simulink model "ariClinderSys"  (R2018a)
settings: Solver=VariableStepAuto  StartTime=0.0  StopTime=10.0  RelTol=1e-3
settings Model: Creator=wangmt  LastModifiedBy=wangmt

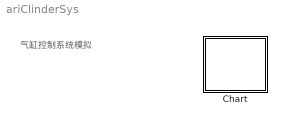
== system ariClinderSys ==
  note: 气缸控制系统模拟
  Chart : Stateflow chart  TreatAsAtomicUnit=on

== stateflow chart ariClinderSys/Chart ==
